simulink model "design_Of_single_phase_cycloconverter"  (R2024a)
settings: Solver=VariableStepAuto  StartTime=0.0  StopTime=0.2  RelTol=1e-3
libraries: spsThyristorLib x8, spsIdealSwitchLib x4, spsRMSLib x2, spsVoltageMeasurementLib x2, spsACVoltageSourceLib x1, spsSeriesRLCBranchLib x1, sps_lib x1
settings Model: Creator=Asus  LastModifiedBy=Asus
settings RTWCC: GPUComputeCapability=3.5

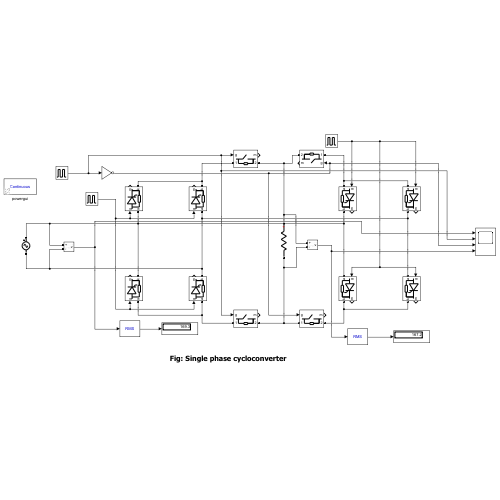
[thumbnail: Simulink's stored preview of the top-level diagram]
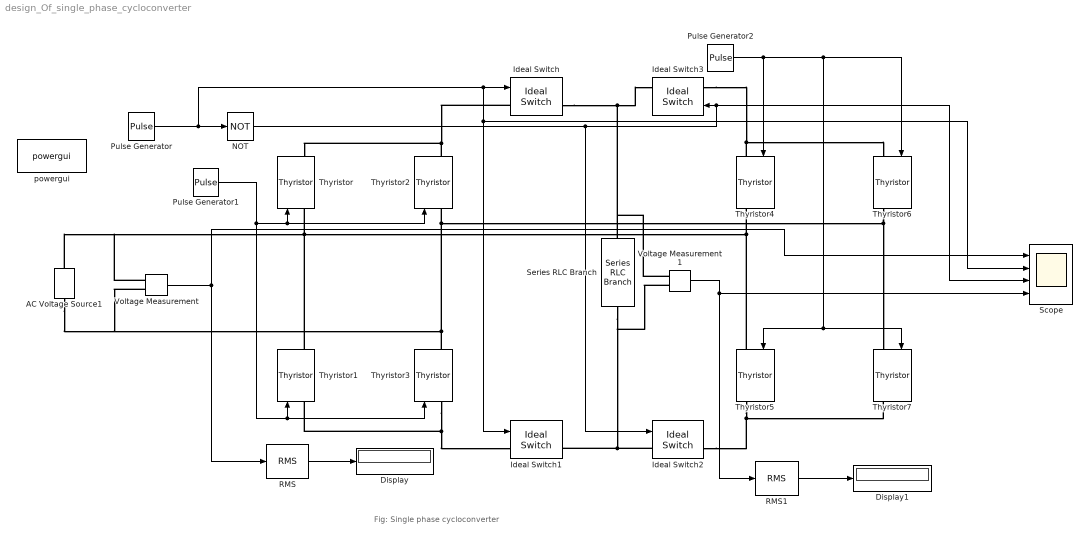
== system design_Of_single_phase_cycloconverter ==
  note: Fig: Single phase cycloconverter
  AC Voltage Source1 : spsACVoltageSourceLib/AC Voltage Source  Amplitude=230  Phase=0  Frequency=50  SampleTime=0  Measurements=None  BusType=swing  Pref=10e3  Qref=0  Qmin=-inf  Qmax=+inf
  Display : Display
  Display1 : Display
  Ideal Switch{,1..3} (4 alike) : spsIdealSwitchLib/Ideal Switch  Ron=0.001  Lon=0  IC=0  Rs=1e5  Cs=inf  Measurements=on
  NOT : Logic  Operator=NOT  IconShape=distinctive  AllPortsSameDT=off  OutDataTypeStr=boolean
  Pulse Generator : DiscretePulseGenerator  PulseType=Time based  Period=0.08  PulseWidth=50
  Pulse Generator1 : DiscretePulseGenerator  PulseType=Time based  Period=.02  PulseWidth=50  PhaseDelay=(30/3600)*0.02
  Pulse Generator2 : DiscretePulseGenerator  PulseType=Time based  Period=10  PulseWidth=5
  RMS : spsRMSLib/RMS  TrueRMS=on  Freq=60  RMSInit=120  Ts=0
  RMS1 : spsRMSLib/RMS  TrueRMS=on  Freq=60  RMSInit=120  Ts=0
  Scope : Scope  NumInputPorts=4
  Series RLC Branch : spsSeriesRLCBranchLib/Series RLC Branch  LConnTagsString=__new0  RConnTagsString=__new0  BranchType=R  Resistance=1  Inductance=1e-3  SetiL0=off  InitialCurrent=0  Capacitance=1e-6  Setx0=off  InitialVoltage=0  Measurements=None
  Thyristor{,1..7} (8 alike) : spsThyristorLib/Thyristor  Ron=0.001  Lon=0  Vf=0.8  IC=0  Rs=500  Cs=250e-9  Measurements=on
  Voltage Measurement : spsVoltageMeasurementLib/Voltage Measurement  PhasorSimulation=off  OutputType=Complex  PSBequivalent=0
  Voltage Measurement1 : spsVoltageMeasurementLib/Voltage Measurement  PhasorSimulation=off  OutputType=Complex  PSBequivalent=0
  powergui : sps_lib/powergui  Priority=1  SimulationMode=Continuous  SampleTime=50e-6  frequency=60  Iterations=50  frequencyindice=50  Pbase=100e6  ErrMax=1e-4  UnitsV=kV  UnitsW=MW  buscounter=0  FunctionMessages=off  echomessages=off  EnableUseOfTLC=off  CurrentSourceSwitches=off  DisableSnubberDevices=off  DisableRonSwitches=off  DisableVfSwitches=off  DisplayEquations=off  AutomaticDiscreteSolvers=off  SolverType=Tustin/Backward Euler (TBE)  Interpol=off  ExternalGateDelay=off  methode=off  Ts=100  x0status=blocks  SPID=on  SwTol=0  HookPort=off  NonlinearTolerance=1e-4  nMaxIteration=100  ContinueOnMaxIteration=off  RestoreLinks=warning  ResistiveCurrentMeasurement=off  Frange=[0:2:500]  Ylog=off  Xlog=on  ShowGrid=off  save=off  variable=ZData  structure=0  ZoomFFT=off  StartTime=0.0  cycles=1  DisplayStyle=1  fundamental=60  FreqAxis=off  MaxFrequency=1000  frequencyindicesteady=1  RmsSteady=1  display=off
  wires:
  Pulse Generator/1 -> Ideal Switch/1, Scope/2, Ideal Switch1/1, NOT/1
  Pulse Generator1/1 -> Thyristor1/1, Thyristor3/1, Thyristor2/1, Thyristor/1
  Pulse Generator2/1 -> Thyristor4/1, Thyristor7/1, Thyristor5/1, Thyristor6/1
  NOT/1 -> Scope/3, Ideal Switch3/1, Ideal Switch2/1
  Voltage Measurement/1 -> Scope/1, RMS/1
  RMS/1 -> Display/1
  RMS1/1 -> Display1/1
  Voltage Measurement1/1 -> Scope/4, RMS1/1
  connections:
  Thyristor2/RConn1 -- Thyristor/RConn1 -- Ideal Switch/LConn1
  Thyristor3/LConn1 -- Ideal Switch1/LConn1 -- Thyristor1/LConn1
  Thyristor1/RConn1 -- Voltage Measurement/LConn1 -- AC Voltage Source1/RConn1 -- Thyristor4/RConn1 -- Thyristor5/LConn1 -- Thyristor/LConn1
  Thyristor4/LConn1 -- Ideal Switch3/LConn1 -- Thyristor6/LConn1
  Thyristor5/RConn1 -- Ideal Switch2/RConn1 -- Thyristor7/RConn1
  Thyristor3/RConn1 -- Thyristor7/LConn1 -- Thyristor6/RConn1 -- Thyristor2/LConn1 -- Voltage Measurement/LConn2 -- AC Voltage Source1/LConn1
  Ideal Switch/RConn1 -- Ideal Switch3/RConn1 -- Voltage Measurement1/LConn1 -- Series RLC Branch/LConn1
  Ideal Switch2/LConn1 -- Voltage Measurement1/LConn2 -- Series RLC Branch/RConn1 -- Ideal Switch1/RConn1
